simulink model "manning_3test_nonlinear"  (R2022b)
settings: Solver=VariableStepAuto  StartTime=0.0  StopTime=5*N  RelTol=1e-3
undefined symbols (not defined in the file or in its folder): yd_ds
settings Model: Creator=chuan  LastModifiedBy=chuan

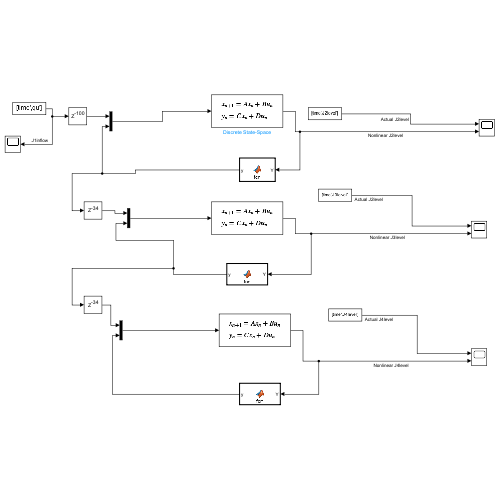
[thumbnail: Simulink's stored preview of the top-level diagram]
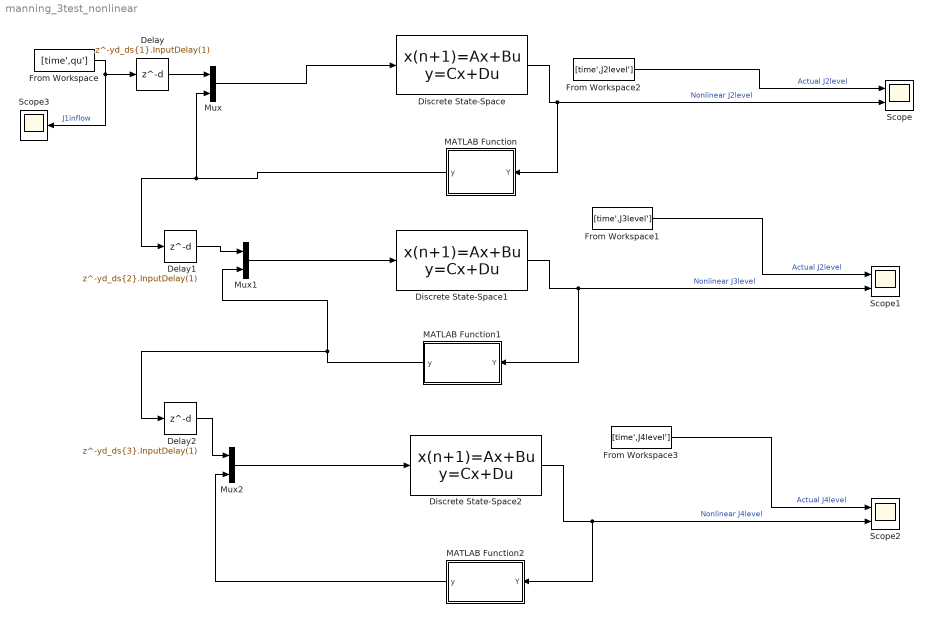
== system manning_3test_nonlinear ==
  Delay : Delay  DelayLength=yd_ds{1}.InputDelay(1)  InitialCondition=0
  Delay1 : Delay  DelayLength=yd_ds{2}.InputDelay(1)  InitialCondition=0
  Delay2 : Delay  DelayLength=yd_ds{3}.InputDelay(1)  InitialCondition=0
  Discrete State-Space : DiscreteStateSpace  A=yd_ds{1}.A  B=yd_ds{1}.B  C=yd_ds{1}.C  D=yd_ds{1}.D  SampleTime=yd_ds{1}.Ts
  Discrete State-Space1 : DiscreteStateSpace  A=yd_ds{2}.A  B=yd_ds{2}.B  C=yd_ds{2}.C  D=yd_ds{2}.D  SampleTime=yd_ds{2}.Ts
  Discrete State-Space2 : DiscreteStateSpace  A=yd_ds{3}.A  B=yd_ds{3}.B  C=yd_ds{3}.C  D=yd_ds{3}.D  SampleTime=yd_ds{3}.Ts
  From Workspace : FromWorkspace  VariableName=[time',qu']
  From Workspace1 : FromWorkspace  VariableName=[time',J3level']
  From Workspace2 : FromWorkspace  VariableName=[time',J2level']
  From Workspace3 : FromWorkspace  VariableName=[time',J4level']
  MATLAB Function : MATLAB Function  TreatAsAtomicUnit=on
  MATLAB Function1 : MATLAB Function  TreatAsAtomicUnit=on
  MATLAB Function2 : MATLAB Function  TreatAsAtomicUnit=on
  Mux : Mux  Inputs=2
  Mux1 : Mux  Inputs=2
  Mux2 : Mux  Inputs=2
  Scope : Scope  NumInputPorts=2
  Scope1 : Scope  NumInputPorts=2
  Scope2 : Scope  NumInputPorts=2
  Scope3 : Scope
  wires:
  Discrete State-Space/1 -> MATLAB Function/1(Y), Scope/2  "Nonlinear J2level"
  Mux/1 -> Discrete State-Space/1
  From Workspace/1 -> Delay/1, Scope3/1  "J1inflow"
  From Workspace2/1 -> Scope/1  "Actual J2level"
  Mux1/1 -> Discrete State-Space1/1
  Discrete State-Space1/1 -> MATLAB Function1/1(Y), Scope1/2  "Nonlinear J3level"
  From Workspace1/1 -> Scope1/1  "Actual J2level"
  Mux2/1 -> Discrete State-Space2/1
  Discrete State-Space2/1 -> MATLAB Function2/1(Y), Scope2/2  "Nonlinear J4level"
  From Workspace3/1 -> Scope2/1  "Actual J4level"
  MATLAB Function/1(y) -> Delay1/1, Mux/2
  MATLAB Function2/1(y) -> Mux2/2
  MATLAB Function1/1(y) -> Delay2/1, Mux1/2
  Delay/1 -> Mux/1
  Delay1/1 -> Mux1/1
  Delay2/1 -> Mux2/1

== matlab function manning_3test_nonlinear/MATLAB Function1 ==
  data: Y input; y output
function y = fcn(Y)
n = 0.03;
Sb = 0.0015;
B= 7;
m = 1.5;

Y = max(Y,0);

y = (1/n)*(B*Y + m*Y.^2)*((B*Y + m*Y.^2)/(B + 2.*Y.*sqrt(1+m^2))).^(2/3) .* sqrt(Sb);

== matlab function manning_3test_nonlinear/MATLAB Function2 ==
  data: Y input; y output
function y = fcn(Y)
n = 0.01;
Sb = 0.0015;
B= 8;
m = 1.5;

Y = max(Y,0);

y = (1/n)*(B*Y + m*Y.^2)*((B*Y + m*Y.^2)/(B + 2.*Y.*sqrt(1+m^2))).^(2/3) .* sqrt(Sb);

== matlab function manning_3test_nonlinear/MATLAB Function ==
  data: Y input; y output
function y = fcn(Y)
n = 0.04;
Sb = 0.0025;
B= 2;
m = 1.5;

Y = max(Y,0);

y = (1/n)*(B*Y + m*Y.^2)*((B*Y + m*Y.^2)/(B + 2.*Y.*sqrt(1+m^2))).^(2/3) .* sqrt(Sb);
